simulink model "NonlinearPendulumModel"  (R2020b)
settings: Solver=VariableStepAuto  StartTime=0.0  StopTime=10.0  RelTol=1e-3
values from neighbouring files (symbols this model uses):
  Bp = 1.4*10^-5    (= 1.4e-05)    [SystemSimulation.m]
  Br = 8.0508*10^-4    (= 0.00080508)    [SystemSimulation.m]
  g = 9.81    [SystemSimulation.m]
  Jp = 1.2551*10^-4    (= 0.00012551)    [SystemSimulation.m]
  Jr = 2.2923*10^-4    (= 0.00022923)    [SystemSimulation.m]
  km = 0.042    [SystemSimulation.m]
  kt = 0.042    [SystemSimulation.m]
  Lp = 0.129    [SystemSimulation.m]
  Lr = 0.085    [SystemSimulation.m]
  mp = 0.024    [SystemSimulation.m]
  Rm = 8.4    [SystemSimulation.m]
  Vlb = -10    [SystemSimulation.m]
  Vub = 10    [SystemSimulation.m]
  x0 = [0 pi 0 0]    [SystemSimulation.m]
settings Model: Creator=Jip  LastModifiedBy=Jip
settings DataIOCC: Refine=10

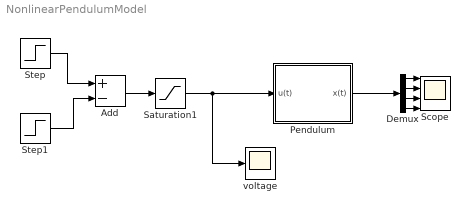
== system NonlinearPendulumModel ==
  Add : Sum  Inputs=+-
  Demux : Demux
  Pendulum : Subsystem
  Saturation1 : Saturate  UpperLimit=Vub  LowerLimit=Vlb
  Scope : Scope  NumInputPorts=4
  Step : Step  Time=0  SampleTime=0
  Step1 : Step  Time=2  After=-1  SampleTime=0
  voltage : Scope
  wires:
  Step/1 -> Add/1
  Saturation1/1 -> Pendulum/1(u(t)), voltage/1
  Pendulum/1(x(t)) -> Demux/1
  Step1/1 -> Add/2
  Add/1 -> Saturation1/1
  Demux/1 -> Scope/1
  Demux/2 -> Scope/2
  Demux/3 -> Scope/3
  Demux/4 -> Scope/4

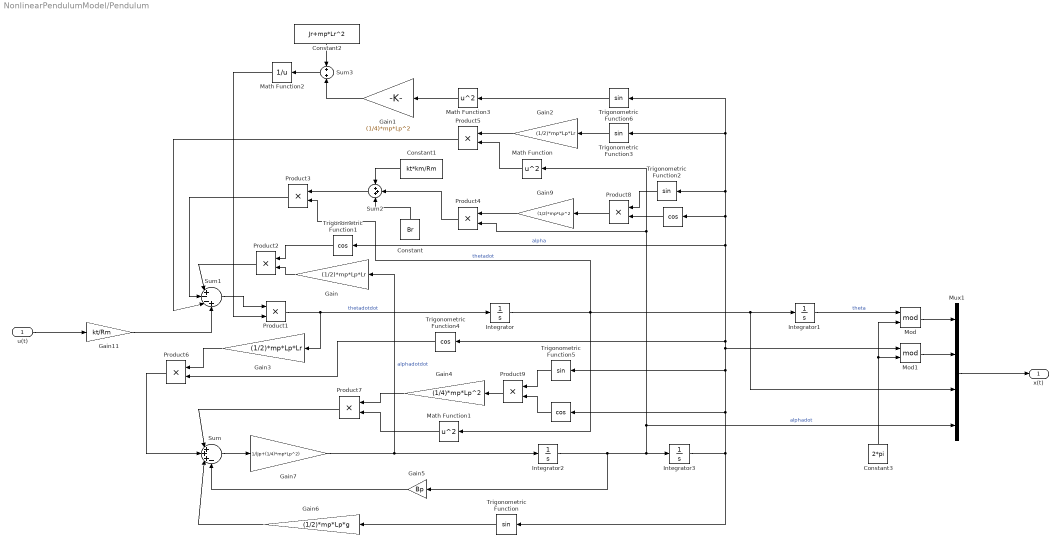
== system NonlinearPendulumModel/Pendulum ==
  u(t) : Inport
  "    " : Trigonometry  Operator=cos
  "     " : Trigonometry  Operator=cos
  Constant : Constant  Value=Br
  Constant1 : Constant  Value=kt*km/Rm
  Constant2 : Constant  Value=Jr+mp*Lr^2
  Constant3 : Constant  Value=2*pi
  Gain : Gain  Gain=(1/2)*mp*Lp*Lr
  Gain1 : Gain  Gain=(1/4)*mp*Lp^2
  Gain11 : Gain  Gain=kt/Rm
  Gain2 : Gain  Gain=(1/2)*mp*Lp*Lr
  Gain3 : Gain  Gain=(1/2)*mp*Lp*Lr
  Gain4 : Gain  Gain=(1/4)*mp*Lp^2
  Gain5 : Gain  Gain=Bp
  Gain6 : Gain  Gain=(1/2)*mp*Lp*g
  Gain7 : Gain  Gain=1/(Jp+(1/4)*mp*Lp^2)
  Gain9 : Gain  Gain=(1/2)*mp*Lp^2
  Integrator : Integrator  InitialCondition=x0(3)
  Integrator1 : Integrator  InitialCondition=x0(1)
  Integrator2 : Integrator  InitialCondition=x0(4)
  Integrator3 : Integrator  InitialCondition=x0(2)
  Math Function : Math  Operator=square  SignedPower=on  SaturateOnIntegerOverflow=on
  Math Function1 : Math  Operator=square  SignedPower=on  SaturateOnIntegerOverflow=on
  Math Function2 : Math  Operator=reciprocal  SignedPower=on  SaturateOnIntegerOverflow=on
  Math Function3 : Math  Operator=square  SignedPower=on  SaturateOnIntegerOverflow=on
  Mod : Math  Operator=mod  SaturateOnIntegerOverflow=on
  Mod1 : Math  Operator=mod  SaturateOnIntegerOverflow=on
  Mux1 : Mux
  Product{1..9} (9 alike) : Product
  Sum : Sum  Inputs=|+++-
  Sum1 : Sum  Inputs=|+--+
  Sum2 : Sum  Inputs=+++
  Sum3 : Sum
  Trigonometric Function{,2..3,5..6} (5 alike) : Trigonometry
  Trigonometric Function1 : Trigonometry  Operator=cos
  Trigonometric Function4 : Trigonometry  Operator=cos
  x(t) : Outport
  wires:
  Trigonometric Function/1 -> Gain6/1
  Gain3/1 -> Product6/1
  Math Function1/1 -> Product7/2
  Gain/1 -> Product2/2
  Integrator1/1 -> Mod/1  "theta"
  Constant1/1 -> Sum2/1
  Gain11/1 -> Sum1/4
  Sum/1 -> Gain7/1
  Gain9/1 -> Product4/1
  Gain7/1 -> Gain/1, Integrator2/1  "alphadotdot"
  Integrator/1 -> Math Function1/1, Product3/2, Mux1/3, Integrator1/1  "thetadot"
  "    "/1 -> Product8/2
  Product9/1 -> Gain4/1
  Product8/1 -> Gain9/1
  "     "/1 -> Product9/2
  Sum1/1 -> Product1/1
  Trigonometric Function3/1 -> Gain2/1
  Product2/1 -> Sum1/1
  Trigonometric Function2/1 -> Product8/1
  Sum2/1 -> Product3/1
  Trigonometric Function4/1 -> Product6/2
  Product6/1 -> Sum/2
  Product7/1 -> Sum/1
  Product3/1 -> Sum1/2
  Gain6/1 -> Sum/3
  Product1/1 -> Gain3/1, Integrator/1  "thetadotdot"
  Integrator3/1 -> Mod1/1, "    "/1, Trigonometric Function2/1, Trigonometric Function6/1, Trigonometric Function3/1, Trigonometric Function1/1, Trigonometric Function4/1, Trigonometric Function5/1, "     "/1, Trigonometric Function/1  "alpha"
  Trigonometric Function5/1 -> Product9/1
  Trigonometric Function1/1 -> Product2/1
  Constant/1 -> Sum2/3
  Product4/1 -> Sum2/2
  Math Function2/1 -> Product1/2
  u(t)/1 -> Gain11/1
  Product5/1 -> Sum1/3
  Integrator2/1 -> Math Function/1, Product4/2, Mux1/4, Integrator3/1, Gain5/1  "alphadot"
  Gain2/1 -> Product5/1
  Gain4/1 -> Product7/1
  Math Function/1 -> Product5/2
  Gain5/1 -> Sum/4
  Mux1/1 -> x(t)/1
  Gain1/1 -> Sum3/2
  Constant2/1 -> Sum3/1
  Sum3/1 -> Math Function2/1
  Trigonometric Function6/1 -> Math Function3/1
  Math Function3/1 -> Gain1/1
  Constant3/1 -> Mod1/2, Mod/2
  Mod/1 -> Mux1/1
  Mod1/1 -> Mux1/2
